simulink subsystem "scale_subsystem"  (R2019b)
settings: Solver=VariableStepAuto  StartTime=0.0  StopTime=10.0  RelTol=1e-3
settings Model: Creator=Matthew  LastModifiedBy=Matthew

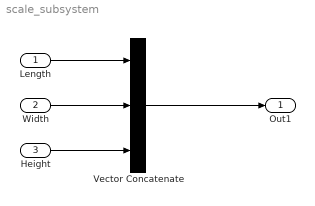
== system scale_subsystem ==
  Length : Inport
  Width : Inport  Port=2
  Height : Inport  Port=3
  Vector Concatenate : Concatenate  NumInputs=3
  Out1 : Outport
  wires:
  Length/1 -> Vector Concatenate/1
  Width/1 -> Vector Concatenate/2
  Height/1 -> Vector Concatenate/3
  Vector Concatenate/1 -> Out1/1
